simulink model "geared_motor_load"  (R2023b)
settings: Solver=VariableStepAuto  StartTime=0.0  StopTime=0.05  RelTol=1e-3
values from neighbouring files (symbols this model uses):
  Beq = Jeq / 0.00376    (= 0.00264630474582)    [homeworktwo.m]
  gain = gear_ratio    (= 0.0123456790123)    [homeworktwo.m]
  gear_alpha = 0.72    [homeworktwo.m]
  gear_ratio = 1/81    (= 0.0123456790123)    [homeworktwo.m]
  Jeq = Jm + (1 / gear_alpha) * gear_ratio * gear_ratio * Jg    (= 9.9501058443e-06)    [homeworktwo.m]
  Ke = 0.0683    [homeworktwo.m]
  Kt = 0.0683    [homeworktwo.m]
  La = 0.000658    [homeworktwo.m]
  Ra = 1.76    [homeworktwo.m]
  Va = 48    [homeworktwo.m]
undefined symbols (not defined in the file or in its folder): Bl, Jl
settings Model: Creator=junseo  LastModifiedBy=minjs
settings OptimizationCC: ReuseModelBlockBuffer=off

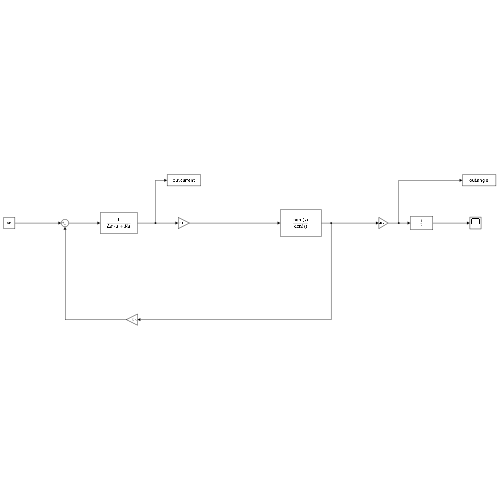
[thumbnail: Simulink's stored preview of the top-level diagram]
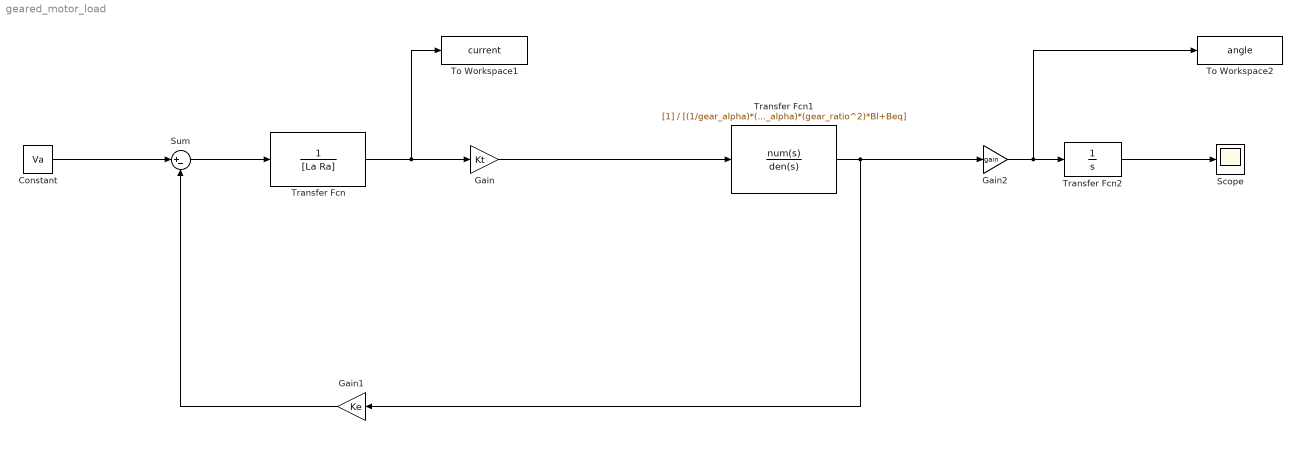
== system geared_motor_load ==
  Constant : Constant  Value=Va
  Gain : Gain  Gain=Kt
  Gain1 : Gain  Gain=Ke
  Gain2 : Gain  Gain=gain
  Scope : Scope
  Sum : Sum  Inputs=|+-
  To Workspace1 : ToWorkspace  VariableName=current  SaveFormat=Timeseries  SampleTime=-1
  To Workspace2 : ToWorkspace  VariableName=angle  SaveFormat=Timeseries  SampleTime=-1
  Transfer Fcn : TransferFcn  Denominator=[La Ra]
  Transfer Fcn1 : TransferFcn  Denominator=[(1/gear_alpha)*(gear_ratio^2)*Jl+Jeq (1/gear_alpha)*(gear_ratio^2)*Bl+Beq]
  Transfer Fcn2 : TransferFcn  Denominator=[1 0]
  wires:
  Constant/1 -> Sum/1
  Sum/1 -> Transfer Fcn/1
  Transfer Fcn/1 -> To Workspace1/1, Gain/1
  Gain/1 -> Transfer Fcn1/1
  Gain1/1 -> Sum/2
  Gain2/1 -> To Workspace2/1, Transfer Fcn2/1
  Transfer Fcn1/1 -> Gain1/1, Gain2/1
  Transfer Fcn2/1 -> Scope/1
